simulink model "PD_gravita"  (R2017b)
settings: Solver=FixedStepAuto  StartTime=0.0  StopTime=40  FixedStep=T  RelTol=1e-3
undefined symbols (not defined in the file or in its folder): DirectDynamicsSim, Gravity, Kd, Kp
settings Model: Creator=Giovanni  LastModifiedBy=Giovanni

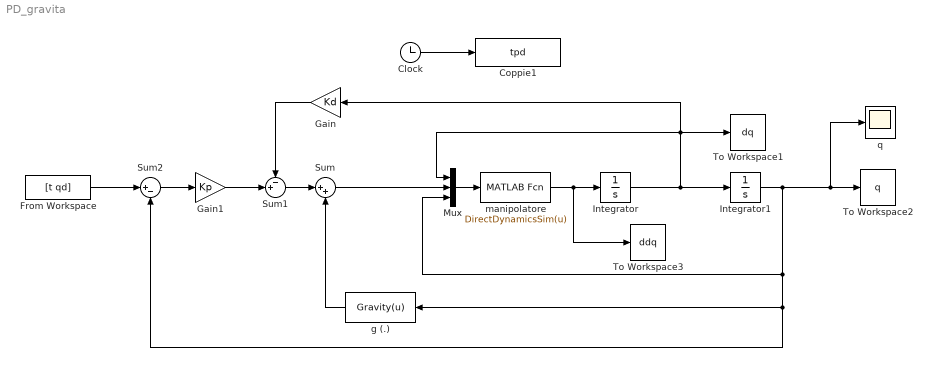
== system PD_gravita ==
  Clock : Clock
  Coppie1 : ToWorkspace  VariableName=tpd  SampleTime=-1
  From Workspace : FromWorkspace  VariableName=[t qd]  SampleTime=0
  Gain : Gain  Gain=Kd
  Gain1 : Gain  Gain=Kp
  Integrator : Integrator  InitialCondition=zeros(6,1)
  Integrator1 : Integrator  InitialCondition=zeros(6,1)
  Mux : Mux  Inputs=3
  Sum : Sum  Inputs=|++
  Sum1 : Sum  Inputs=-+|
  Sum2 : Sum  Inputs=|+-
  To Workspace1 : ToWorkspace  VariableName=dq  SampleTime=-1
  To Workspace2 : ToWorkspace  VariableName=q  SampleTime=-1
  To Workspace3 : ToWorkspace  VariableName=ddq  SampleTime=-1
  g (.) : MATLABFcn  MATLABFcn=Gravity(u)
  manipolatore : MATLABFcn  MATLABFcn=DirectDynamicsSim(u)
  q : Scope
  wires:
  Clock/1 -> Coppie1/1
  manipolatore/1 -> To Workspace3/1, Integrator/1
  Integrator1/1 -> q/1, To Workspace2/1, Sum2/2, g (.)/1, Mux/3
  Integrator/1 -> Integrator1/1, Gain/1, Mux/1, To Workspace1/1
  Mux/1 -> manipolatore/1
  Sum/1 -> Mux/2
  g (.)/1 -> Sum/2
  Sum1/1 -> Sum/1
  Gain/1 -> Sum1/1
  Gain1/1 -> Sum1/2
  Sum2/1 -> Gain1/1
  From Workspace/1 -> Sum2/1
